simulink model "main"  (R2023b)
settings: Solver=ode113  StartTime=tstart  StopTime=tend  RelTol=relTol  AbsTol=absTol
values from neighbouring files (symbols this model uses):
  D_init = JD_init - 2451545.0    (= 1484.5)    [EulerEquations.m]    (also in main_script.m)
  DCM_initial = targetDCM([26321453.5527815,	-132781955.130633,	-57571626.5531097]', R_princ)    [EulerEquations.m]    (also in main_script.m)
  EKF_P0 = eye(7)    [main_script.m]
  EKF_x0 = [0,0,0,0,0,0,0]    [main_script.m]
  inertia_p = [85.075, 0, 0; 0, 85.075, 0; 0, 0, 120.2515]    [omega_dot.m]
  omega_init = [0; 0; 0.01]    [EulerEquations.m]    (also in main_script.m = [0; 0; 0.0])
  state_ECI_init = [R_PQW_IJK*state_PQW_init(1:3)';R_PQW_IJK*state_PQW_init(4:6)']    [OrbitPropagation.m]
  theta = UT1_to_theta(UT1)    [EulerEquations.m]    (also in UT1_to_theta.m = rotz(-GMST*180/pi); main_script.m)
  tstart = 0    [EulerEquations.m]    (also in main_script.m)
  UT1 = [1,25,2004,00]    [EulerEquations.m]    (also in main_script.m)
undefined symbols (not defined in the file or in its folder): a_sun, e_sun, i_sun, M0_sun, n_sun, Om_sun, om_sun, R_princ
libraries: dspmathops x2, aerolibatmos2 x1, simulink x1, matrix_library x1
(part 1 of 2)
settings Model: Creator=Anna  LastModifiedBy=Anna

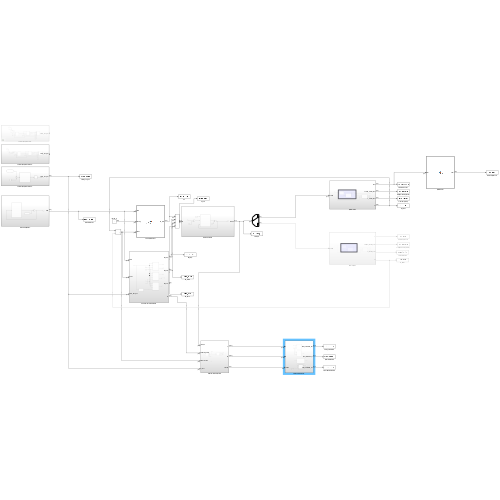
[thumbnail: Simulink's stored preview of the top-level diagram]
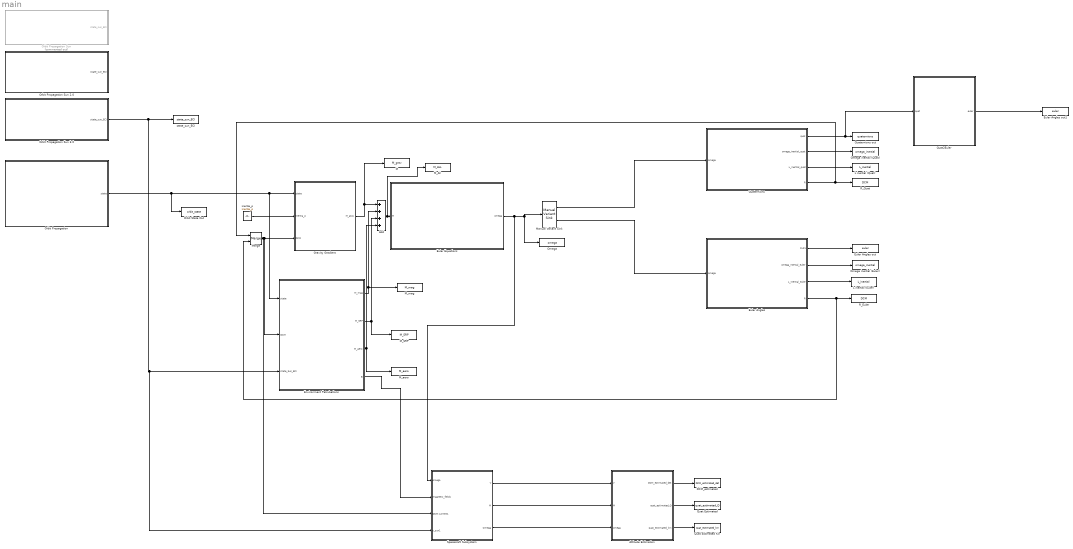
== system main ==
  Add : Sum  Inputs=++++
  Attitude Estimation : Subsystem
  DCM_estimated : ToWorkspace  VariableName=DCM_estimated_det  SaveFormat=Timeseries  SampleTime=-1
      settings: Save2DSignal=2-D array (concatenate along first dimension)
  Environment Petrubations : Subsystem
  Euler Angles : Subsystem
  Euler Angles out : ToWorkspace  VariableName=euler  SaveFormat=Timeseries  SampleTime=-1
  Euler Angles out1 : ToWorkspace  VariableName=euler  SaveFormat=Timeseries  SampleTime=-1
  Euler Equations : Subsystem
  Gravity Gradient : MATLAB Function  TreatAsAtomicUnit=on
  L inertial (Euler) : ToWorkspace  VariableName=L_inertial  SaveFormat=Timeseries  SampleTime=-1
  L inertial (Quat) : ToWorkspace  VariableName=L_inertial  SaveFormat=Timeseries  SampleTime=-1
  M : ToWorkspace  VariableName=M_grav  SaveFormat=Timeseries  SampleTime=-1
      settings: Save2DSignal=2-D array (concatenate along first dimension)
  M_All : ToWorkspace  VariableName=M_ALL  SaveFormat=Timeseries  SampleTime=-1
      settings: Save2DSignal=2-D array (concatenate along first dimension)
  M_SRP : ToWorkspace  VariableName=M_SRP  SaveFormat=Timeseries  SampleTime=-1
      settings: Save2DSignal=2-D array (concatenate along first dimension)
  M_aero : ToWorkspace  VariableName=M_aero  SaveFormat=Timeseries  SampleTime=-1
      settings: Save2DSignal=2-D array (concatenate along first dimension)
  M_mag : ToWorkspace  VariableName=M_mag  SaveFormat=Timeseries  SampleTime=-1
      settings: Save2DSignal=2-D array (concatenate along first dimension)
  Manual Variant Sink : simulink/Signal Routing/Manual Variant Sink  NumChoices=2  LabelModeActiveChoice=V_1
  Merge : Merge
  Omega : ToWorkspace  VariableName=omega  SaveFormat=Timeseries  SampleTime=-1
      settings: Save2DSignal=2-D array (concatenate along first dimension)
  Omega inertial (Euler) : ToWorkspace  VariableName=omega_inertial  SaveFormat=Timeseries  SampleTime=-1
  Omega inertial (Quat) : ToWorkspace  VariableName=omega_inertial  SaveFormat=Timeseries  SampleTime=-1
  Orbit Propagation : Subsystem
  Orbit Propagation Sun : Subsystem  Commented=on
  Orbit Propagation Sun 2.0 : Subsystem
  Orbit Propagation Sun 3.0 : Subsystem
  Orbit State Out : ToWorkspace  VariableName=orbit_state  SaveFormat=Timeseries  SampleTime=-1
  Quat Estimated : ToWorkspace  VariableName=quat_estimated_Q  SaveFormat=Timeseries  SampleTime=-1
  Quat Estimated Kin : ToWorkspace  VariableName=quat_estimated_kin  SaveFormat=Timeseries  SampleTime=-1
  Quat2Euler : MATLAB Function  TreatAsAtomicUnit=on
  Quaternions : Subsystem
  Quaternions out : ToWorkspace  VariableName=quaternions  SaveFormat=Timeseries  SampleTime=-1
  R_Euler : ToWorkspace  VariableName=DCM  SaveFormat=Timeseries  SampleTime=-1
  R_Quat : ToWorkspace  VariableName=DCM  SaveFormat=Timeseries  SampleTime=-1
  Spacecraft Subsystem : Subsystem
  inertia_p : Constant  Value=inertia_p
  state_sun_ECI : ToWorkspace  VariableName=state_sun_ECI  SaveFormat=Timeseries  SampleTime=-1
  wires:
  Quaternions/1(quat) -> Quat2Euler/1(quat), Quaternions out/1
  Quaternions/2(omega_inertial_quat) -> Omega inertial (Quat)/1
  Quaternions/3(L_inertial_quat) -> L inertial (Quat)/1
  Quaternions/4(R) -> Merge/1, R_Quat/1
  Euler Angles/1(Out1) -> Euler Angles out/1
  Euler Angles/2(omega_inertial_euler) -> Omega inertial (Euler)/1
  Euler Angles/3(L_inertial_euler) -> L inertial (Euler)/1
  Euler Angles/4(R) -> Merge/2, R_Euler/1
  Manual Variant Sink/2 -> Euler Angles/1(omega)
  Euler Equations/1(omega) -> Spacecraft Subsystem/1(omega), Manual Variant Sink/1, Omega/1
  Manual Variant Sink/1 -> Quaternions/1(omega)
  Gravity Gradient/1(M_grav) -> Add/1, M/1
  inertia_p/1 -> Gravity Gradient/2(inertia_p)
  Orbit Propagation/1(state) -> Orbit State Out/1, Gravity Gradient/1(state), Environment Petrubations/1(state)
  Quat2Euler/1(euler) -> Euler Angles out1/1
  Merge/1 -> Spacecraft Subsystem/3(DCM current1), Gravity Gradient/3(DCM), Environment Petrubations/2(DCM)
  Add/1 -> M_All/1, Euler Equations/1(M)
  Environment Petrubations/1(M_mag) -> M_mag/1, Add/2
  Environment Petrubations/2(M_SRP) -> M_SRP/1, Add/3
  Environment Petrubations/3(M_aero) -> M_aero/1, Add/4
  Orbit Propagation Sun 3.0/1(state_sun_ECI) -> state_sun_ECI/1, Environment Petrubations/3(state_Sun_ECI), Spacecraft Subsystem/4(r_sun1)
  Spacecraft Subsystem/1(V) -> Attitude Estimation/1(V)
  Spacecraft Subsystem/2(M) -> Attitude Estimation/2(M)
  Environment Petrubations/4(B) -> Spacecraft Subsystem/2(magnetic_field1)
  Attitude Estimation/1(DCM_estimated_det) -> DCM_estimated/1
  Attitude Estimation/2(quat_estimated_Q) -> Quat Estimated/1
  Attitude Estimation/3(quat_estimated_kin) -> Quat Estimated Kin/1
  Spacecraft Subsystem/3(Omega) -> Attitude Estimation/3(omega)

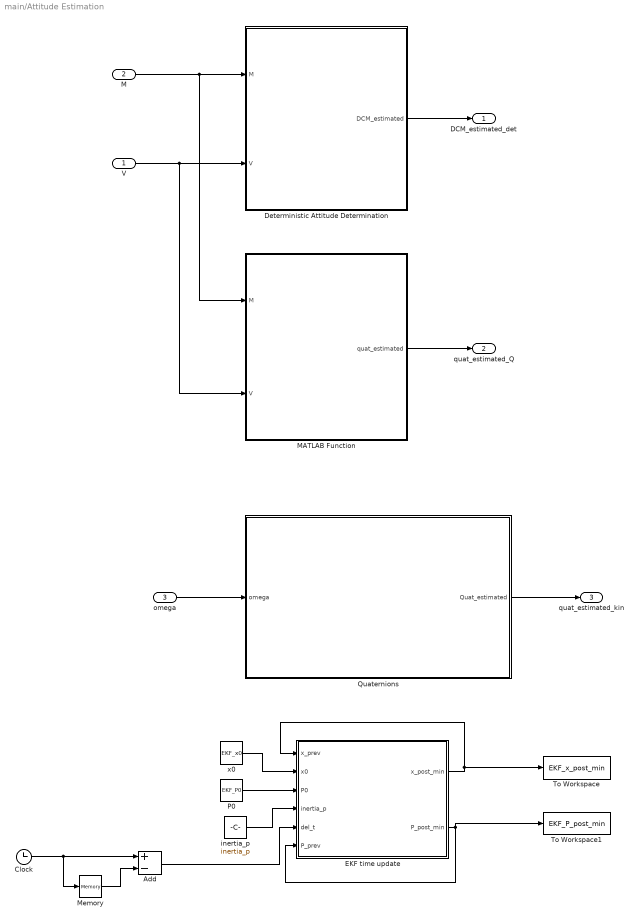
== system main/Attitude Estimation ==
  V : Inport
  M : Inport  Port=2
  omega : Inport  Port=3
  Add : Sum  Inputs=+-
  Clock : Clock
  Deterministic Attitude Determination : MATLAB Function  TreatAsAtomicUnit=on
  EKF time update : MATLAB Function  TreatAsAtomicUnit=on
  MATLAB Function : MATLAB Function  TreatAsAtomicUnit=on
  Memory : Memory
  P0 : Constant  Value=EKF_P0
  Quaternions : Subsystem
  To Workspace : ToWorkspace  VariableName=EKF_x_post_min  SaveFormat=Timeseries  SampleTime=-1
  To Workspace1 : ToWorkspace  VariableName=EKF_P_post_min  SaveFormat=Timeseries  SampleTime=-1
  inertia_p : Constant  Value=inertia_p
  x0 : Constant  Value=EKF_x0
  DCM_estimated_det : Outport
  quat_estimated_Q : Outport  Port=2
  quat_estimated_kin : Outport  Port=3
  wires:
  Deterministic Attitude Determination/1(DCM_estimated) -> DCM_estimated_det/1
  MATLAB Function/1(quat_estimated) -> quat_estimated_Q/1
  M/1 -> MATLAB Function/1(M), Deterministic Attitude Determination/1(M)
  Quaternions/1(Quat_estimated) -> quat_estimated_kin/1
  V/1 -> MATLAB Function/2(V), Deterministic Attitude Determination/2(V)
  omega/1 -> Quaternions/1(omega)
  EKF time update/1(x_post_min) -> To Workspace/1, EKF time update/1(x_prev)
  EKF time update/2(P_post_min) -> To Workspace1/1, EKF time update/6(P_prev)
  x0/1 -> EKF time update/2(x0)
  P0/1 -> EKF time update/3(P0)
  inertia_p/1 -> EKF time update/4(inertia_p)
  Add/1 -> EKF time update/5(del_t)
  Memory/1 -> Add/2
  Clock/1 -> Memory/1, Add/1

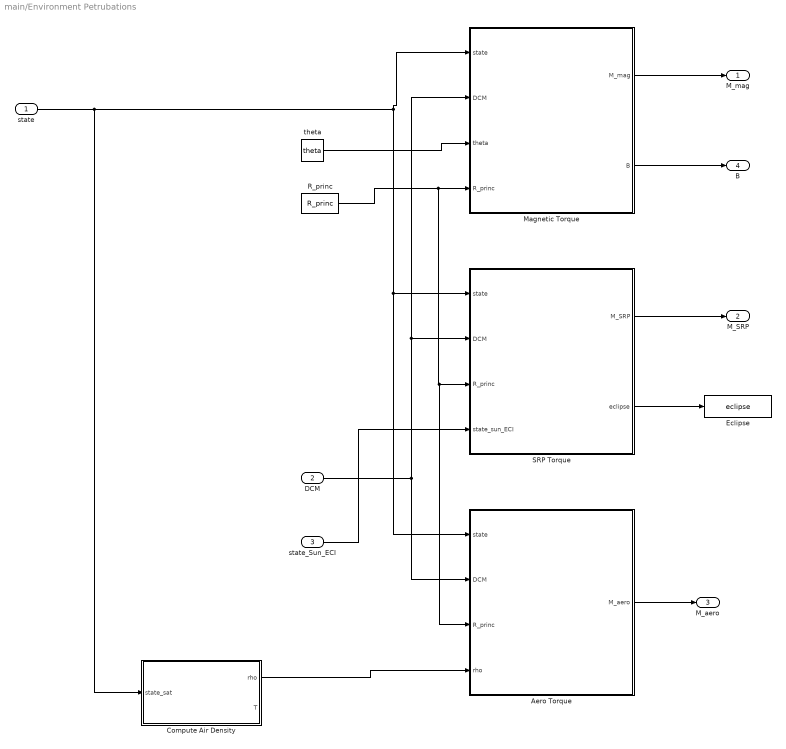
== system main/Environment Petrubations ==
  state : Inport
  DCM : Inport  Port=2
  state_Sun_ECI : Inport  Port=3
  Aero Torque : MATLAB Function  TreatAsAtomicUnit=on
  Compute Air Density : Subsystem
  Eclipse : ToWorkspace  VariableName=eclipse  SaveFormat=Timeseries  SampleTime=-1
  Magnetic Torque : MATLAB Function  TreatAsAtomicUnit=on
  R_princ : Constant  Value=R_princ
  SRP Torque : MATLAB Function  TreatAsAtomicUnit=on
  theta : Constant  Value=theta
  M_mag : Outport
  M_SRP : Outport  Port=2
  M_aero : Outport  Port=3
  B : Outport  Port=4
  wires:
  Magnetic Torque/1(M_mag) -> M_mag/1
  SRP Torque/1(M_SRP) -> M_SRP/1
  state/1 -> Compute Air Density/1(state_sat), Magnetic Torque/1(state), Aero Torque/1(state), SRP Torque/1(state)
  DCM/1 -> Aero Torque/2(DCM), Magnetic Torque/2(DCM), SRP Torque/2(DCM)
  theta/1 -> Magnetic Torque/3(theta)
  R_princ/1 -> Aero Torque/3(R_princ), SRP Torque/3(R_princ), Magnetic Torque/4(R_princ)
  state_Sun_ECI/1 -> SRP Torque/4(state_sun_ECI)
  Aero Torque/1(M_aero) -> M_aero/1
  Compute Air Density/1(rho) -> Aero Torque/4(rho)
  SRP Torque/2(eclipse) -> Eclipse/1
  Magnetic Torque/2(B) -> B/1

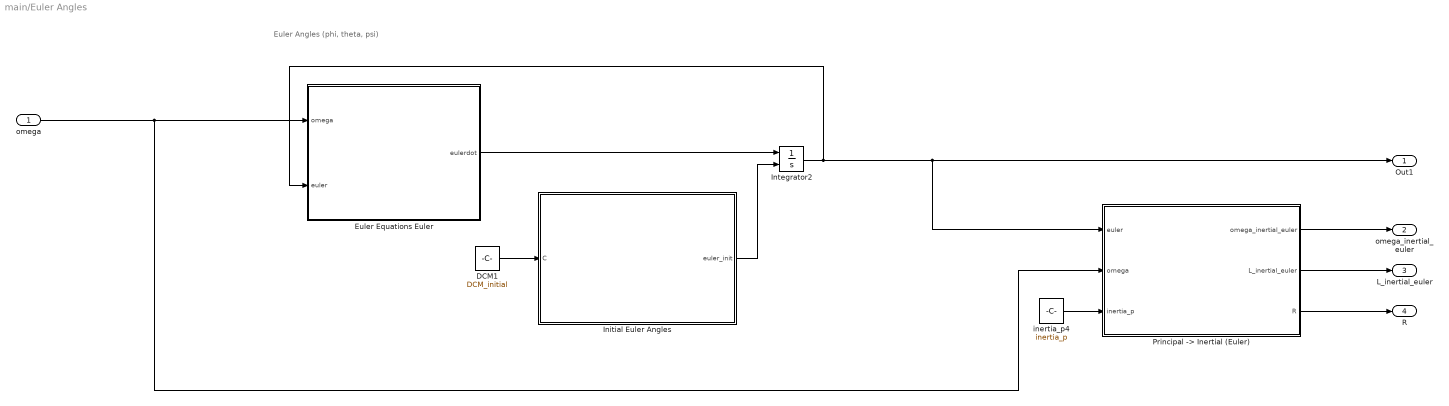
== system main/Euler Angles ==
  note: Euler Angles (phi, theta, psi)
  omega : Inport
  DCM1 : Constant  Value=DCM_initial
  Euler Equations Euler : MATLAB Function  TreatAsAtomicUnit=on
  Initial Euler Angles : MATLAB Function  TreatAsAtomicUnit=on
  Integrator2 : Integrator  InitialConditionSource=external  AbsoluteTolerance=absTol
  "Principal -> Inertial (Euler)" : MATLAB Function  TreatAsAtomicUnit=on
  inertia_p4 : Constant  Value=inertia_p
  Out1 : Outport
  omega_inertial_euler : Outport  Port=2
  L_inertial_euler : Outport  Port=3
  R : Outport  Port=4
  wires:
  "Principal -> Inertial (Euler)"/2(L_inertial_euler) -> L_inertial_euler/1
  Initial Euler Angles/1(euler_init) -> Integrator2/2
  "Principal -> Inertial (Euler)"/1(omega_inertial_euler) -> omega_inertial_euler/1
  "Principal -> Inertial (Euler)"/3(R) -> R/1
  Integrator2/1 -> Out1/1, "Principal -> Inertial (Euler)"/1(euler), Euler Equations Euler/2(euler)
  Euler Equations Euler/1(eulerdot) -> Integrator2/1
  omega/1 -> "Principal -> Inertial (Euler)"/2(omega), Euler Equations Euler/1(omega)
  inertia_p4/1 -> "Principal -> Inertial (Euler)"/3(inertia_p)
  DCM1/1 -> Initial Euler Angles/1(C)

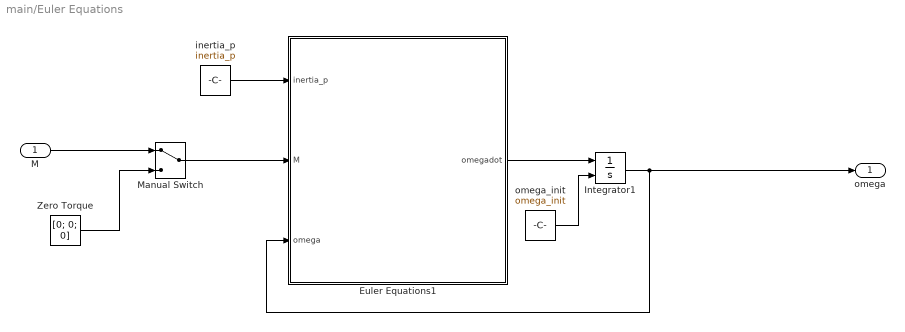
== system main/Euler Equations ==
  M : Inport
  Euler Equations1 : MATLAB Function  TreatAsAtomicUnit=on
  Integrator1 : Integrator  InitialConditionSource=external  AbsoluteTolerance=absTol
  Manual Switch : ManualSwitch
  Zero Torque : Constant  Value=[0; 0; 0]
  inertia_p : Constant  Value=inertia_p
  omega_init : Constant  Value=omega_init
  omega : Outport
  wires:
  inertia_p/1 -> Euler Equations1/1(inertia_p)
  Euler Equations1/1(omegadot) -> Integrator1/1
  Integrator1/1 -> omega/1, Euler Equations1/3(omega)
  omega_init/1 -> Integrator1/2
  Manual Switch/1 -> Euler Equations1/2(M)
  M/1 -> Manual Switch/1
  Zero Torque/1 -> Manual Switch/2

== system main/Orbit Propagation ==
  Integrator3 : Integrator  InitialConditionSource=external  AbsoluteTolerance=absTol
  Orbit Propagation1 : MATLAB Function  TreatAsAtomicUnit=on
  initial state ECI : Constant  Value=state_ECI_init
  state : Outport
  wires:
  initial state ECI/1 -> Integrator3/2
  Orbit Propagation1/1(statedot) -> Integrator3/1
  Integrator3/1 -> state/1, Orbit Propagation1/1(state)

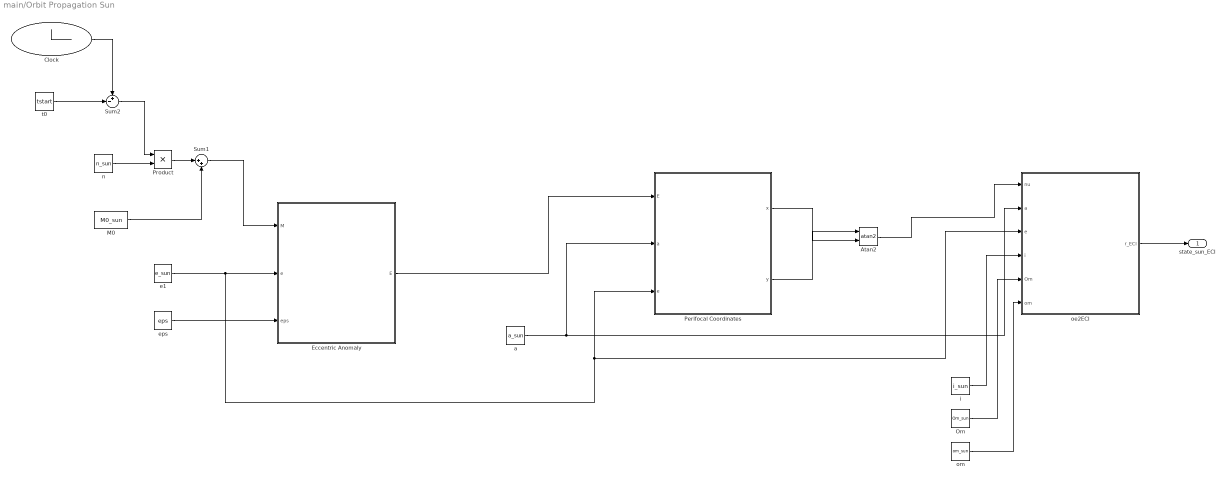
== system main/Orbit Propagation Sun ==
  Atan2 : Trigonometry  Operator=atan2
  Clock : Clock
  Eccentric Anomaly : MATLAB Function  TreatAsAtomicUnit=on
  M0 : Constant  Value=M0_sun
  Om : Constant  Value=Om_sun
  Perifocal Coordinates : MATLAB Function  TreatAsAtomicUnit=on
  Product : Product
  Sum1 : Sum  Inputs=|++
  Sum2 : Sum  Inputs=+-|
  a : Constant  Value=a_sun
  e1 : Constant  Value=e_sun
  eps : Constant  Value=eps
  i : Constant  Value=i_sun
  n : Constant  Value=n_sun
  oe2ECI : MATLAB Function  TreatAsAtomicUnit=on
  om : Constant  Value=om_sun
  t0 : Constant  Value=tstart
  state_sun_ECI : Outport
  wires:
  oe2ECI/1(r_ECI) -> state_sun_ECI/1
  Om/1 -> oe2ECI/5(Om)
  Perifocal Coordinates/2(y) -> Atan2/1
  Perifocal Coordinates/1(x) -> Atan2/2
  i/1 -> oe2ECI/4(i)
  Atan2/1 -> oe2ECI/1(nu)
  e1/1 -> oe2ECI/3(e), Perifocal Coordinates/3(e), Eccentric Anomaly/2(e)
  a/1 -> Perifocal Coordinates/2(a), oe2ECI/2(a)
  om/1 -> oe2ECI/6(om)
  eps/1 -> Eccentric Anomaly/3(eps)
  Eccentric Anomaly/1(E) -> Perifocal Coordinates/1(E)
  Sum1/1 -> Eccentric Anomaly/1(M)
  M0/1 -> Sum1/2
  Sum2/1 -> Product/1
  Clock/1 -> Sum2/1
  n/1 -> Product/2
  Product/1 -> Sum1/1
  t0/1 -> Sum2/2

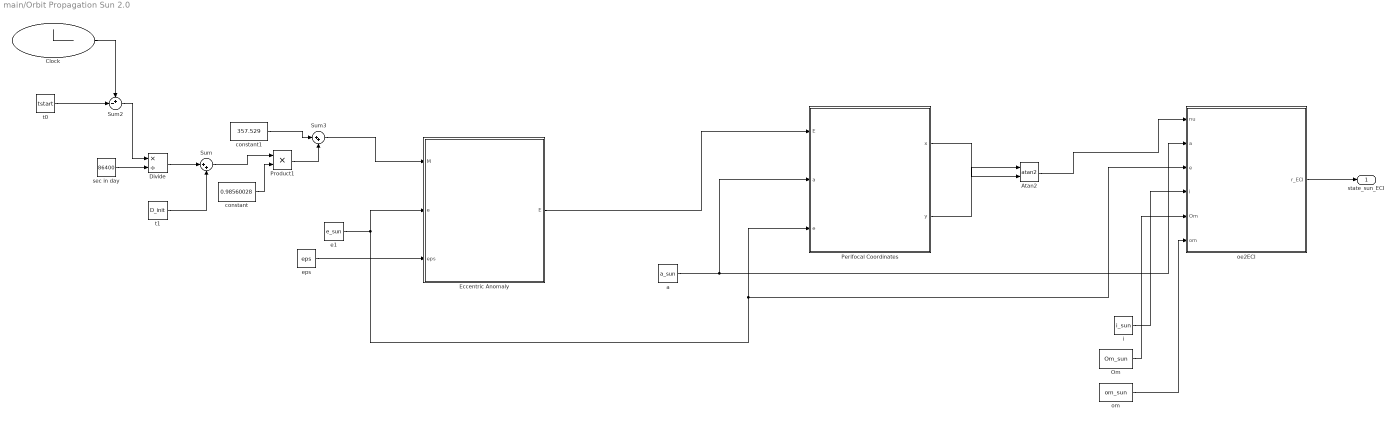
== system main/Orbit Propagation Sun 2.0 ==
  Atan2 : Trigonometry  Operator=atan2
  Clock : Clock
  Divide : Product  Inputs=*/
  Eccentric Anomaly : MATLAB Function  TreatAsAtomicUnit=on
  Om : Constant  Value=Om_sun
  Perifocal Coordinates : MATLAB Function  TreatAsAtomicUnit=on
  Product1 : Product
  Sum : Sum  Inputs=|++
  Sum2 : Sum  Inputs=+-|
  Sum3 : Sum  Inputs=|++
  a : Constant  Value=a_sun
  constant : Constant  Value=0.98560028
  constant1 : Constant  Value=357.529
  e1 : Constant  Value=e_sun
  eps : Constant  Value=eps
  i : Constant  Value=i_sun
  oe2ECI : MATLAB Function  TreatAsAtomicUnit=on
  om : Constant  Value=om_sun
  sec in day : Constant  Value=86400
  t0 : Constant  Value=tstart
  t1 : Constant  Value=D_init
  state_sun_ECI : Outport
  wires:
  oe2ECI/1(r_ECI) -> state_sun_ECI/1
  Om/1 -> oe2ECI/5(Om)
  Perifocal Coordinates/2(y) -> Atan2/1
  Perifocal Coordinates/1(x) -> Atan2/2
  i/1 -> oe2ECI/4(i)
  Atan2/1 -> oe2ECI/1(nu)
  e1/1 -> Eccentric Anomaly/2(e), oe2ECI/3(e), Perifocal Coordinates/3(e)
  a/1 -> Perifocal Coordinates/2(a), oe2ECI/2(a)
  om/1 -> oe2ECI/6(om)
  eps/1 -> Eccentric Anomaly/3(eps)
  Eccentric Anomaly/1(E) -> Perifocal Coordinates/1(E)
  Clock/1 -> Sum2/1
  t0/1 -> Sum2/2
  Sum2/1 -> Divide/1
  sec in day/1 -> Divide/2
  Divide/1 -> Sum/1
  t1/1 -> Sum/2
  Sum/1 -> Product1/1
  constant/1 -> Product1/2
  Product1/1 -> Sum3/2
  constant1/1 -> Sum3/1
  Sum3/1 -> Eccentric Anomaly/1(M)

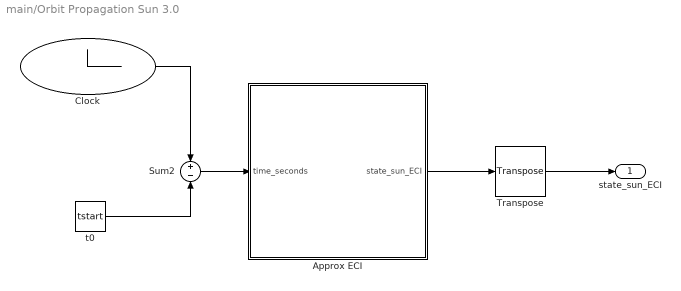
== system main/Orbit Propagation Sun 3.0 ==
  Approx ECI : MATLAB Function  TreatAsAtomicUnit=on
  Clock : Clock
  Sum2 : Sum  Inputs=+-
  Transpose : matrix_library/Transpose
  t0 : Constant  Value=tstart
  state_sun_ECI : Outport
  wires:
  Clock/1 -> Sum2/1
  t0/1 -> Sum2/2
  Sum2/1 -> Approx ECI/1(time_seconds)
  Transpose/1 -> state_sun_ECI/1
  Approx ECI/1(state_sun_ECI) -> Transpose/1

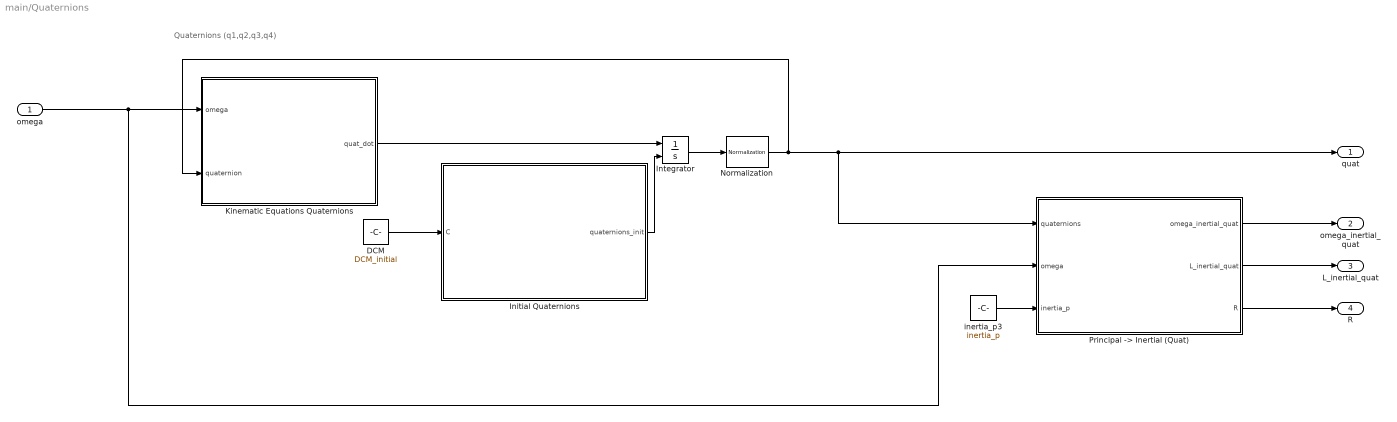
== system main/Quaternions ==
  note: Quaternions (q1,q2,q3,q4)
  omega : Inport
  DCM : Constant  Value=DCM_initial
  Initial Quaternions : MATLAB Function  TreatAsAtomicUnit=on
  Integrator : Integrator  InitialConditionSource=external  AbsoluteTolerance=absTol
  "Kinematic Equations Quaternions " : MATLAB Function  TreatAsAtomicUnit=on
  Normalization : dspmathops/Normalization  NormType=Squared 2-norm  Bias=1e-10  NormOver=Each column  Dimension=1  roundingMode=Floor  overflowMode=off  accumDataTypeStr=Inherit: Same as product output  accumLastDataTypeStr=Inherit: Same as product output  outputDataTypeStr=Inherit: Same as product output  outputMin=[]  outputMax=[]  outputLastDataTypeStr=Inherit: Same as product output
  "Principal -> Inertial (Quat)" : MATLAB Function  TreatAsAtomicUnit=on
  inertia_p3 : Constant  Value=inertia_p
  quat : Outport
  omega_inertial_quat : Outport  Port=2
  L_inertial_quat : Outport  Port=3
  R : Outport  Port=4
  wires:
  omega/1 -> "Kinematic Equations Quaternions "/1(omega), "Principal -> Inertial (Quat)"/2(omega)
  DCM/1 -> Initial Quaternions/1(C)
  "Principal -> Inertial (Quat)"/2(L_inertial_quat) -> L_inertial_quat/1
  "Kinematic Equations Quaternions "/1(quat_dot) -> Integrator/1
  "Principal -> Inertial (Quat)"/3(R) -> R/1
  Initial Quaternions/1(quaternions_init) -> Integrator/2
  Integrator/1 -> Normalization/1
  inertia_p3/1 -> "Principal -> Inertial (Quat)"/3(inertia_p)
  "Principal -> Inertial (Quat)"/1(omega_inertial_quat) -> omega_inertial_quat/1
  Normalization/1 -> quat/1, "Principal -> Inertial (Quat)"/1(quaternions), "Kinematic Equations Quaternions "/2(quaternion)

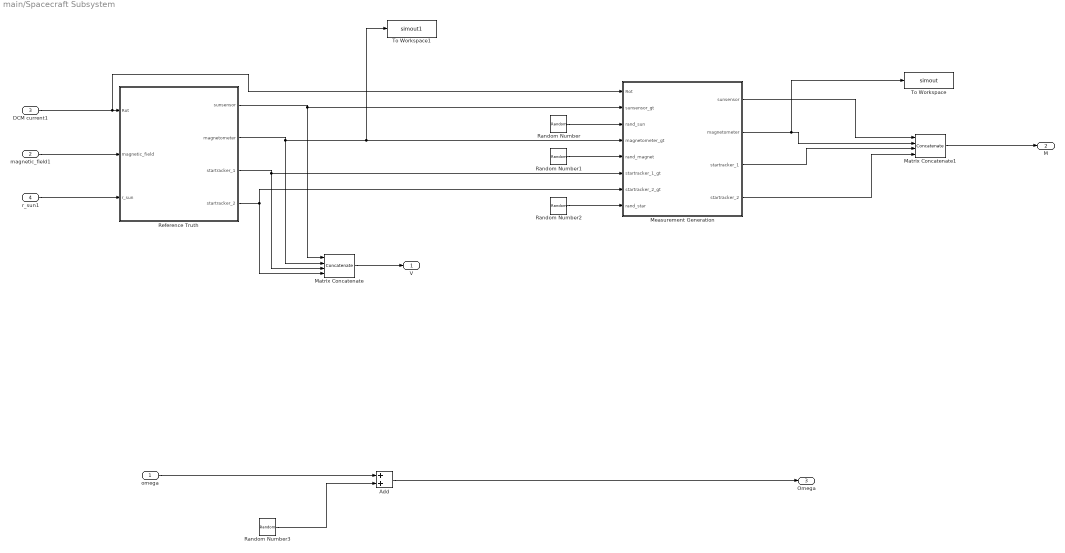
== system main/Spacecraft Subsystem ==
  omega : Inport
  magnetic_field1 : Inport  Port=2
  DCM current1 : Inport  Port=3
  r_sun1 : Inport  Port=4
  Add : Sum
  Matrix Concatenate : Concatenate  NumInputs=4  Mode=Multidimensional array  ConcatenateDimension=2
  Matrix Concatenate1 : Concatenate  NumInputs=4  Mode=Multidimensional array  ConcatenateDimension=2
  Measurement Generation : MATLAB Function  TreatAsAtomicUnit=on
  Random Number : RandomNumber  Variance=0.01  Seed=[80, 81]  SampleTime=0.1
  Random Number1 : RandomNumber  Variance=0.0075*0.000065  Seed=[70, 71, 72]  SampleTime=0.1
  Random Number2 : RandomNumber  Variance=(5/3600)  Seed=[0, 1,2,3,4,5,6,7,8,9,10,11,12,13,14; 15,16,17,18,19,20,21,22,23,24,25,26,27,28,29; 30, 31, 32,33,34,35,36,37,38,39,40,41,42,43,44;45,46,47,48,49,50,51,52,53,54,55,56,57,58,59]  SampleTime=0.1
  Random Number3 : RandomNumber  Variance=0.005  Seed=[101, 102, 103]  SampleTime=0.1
  Reference Truth : MATLAB Function  TreatAsAtomicUnit=on
  To Workspace : ToWorkspace  VariableName=simout  SaveFormat=Timeseries  SampleTime=-1
  To Workspace1 : ToWorkspace  VariableName=simout1  SaveFormat=Timeseries  SampleTime=-1
  V : Outport
  M : Outport  Port=2
  Omega : Outport  Port=3
  wires:
  r_sun1/1 -> Reference Truth/3(r_sun)
  magnetic_field1/1 -> Reference Truth/2(magnetic_field)
  DCM current1/1 -> Measurement Generation/1(Rot), Reference Truth/1(Rot)
  Matrix Concatenate1/1 -> M/1
  Matrix Concatenate/1 -> V/1
  Reference Truth/1(sunsensor) -> Matrix Concatenate/1, Measurement Generation/2(sunsensor_gt)
  Reference Truth/3(startracker_1) -> Measurement Generation/6(startracker_1_gt), Matrix Concatenate/3
  Reference Truth/4(startracker_2) -> Measurement Generation/7(startracker_2_gt), Matrix Concatenate/4
  Measurement Generation/1(sunsensor) -> Matrix Concatenate1/1
  Random Number/1 -> Measurement Generation/3(rand_sun)
  Random Number1/1 -> Measurement Generation/5(rand_magnet)
  Random Number2/1 -> Measurement Generation/8(rand_star)
  Measurement Generation/2(magnetometer) -> To Workspace/1, Matrix Concatenate1/2
  Measurement Generation/4(startracker_2) -> Matrix Concatenate1/4
  Reference Truth/2(magnetometer) -> To Workspace1/1, Measurement Generation/4(magnetometer_gt), Matrix Concatenate/2
  Measurement Generation/3(startracker_1) -> Matrix Concatenate1/3
  omega/1 -> Add/1
  Random Number3/1 -> Add/2
  Add/1 -> Omega/1

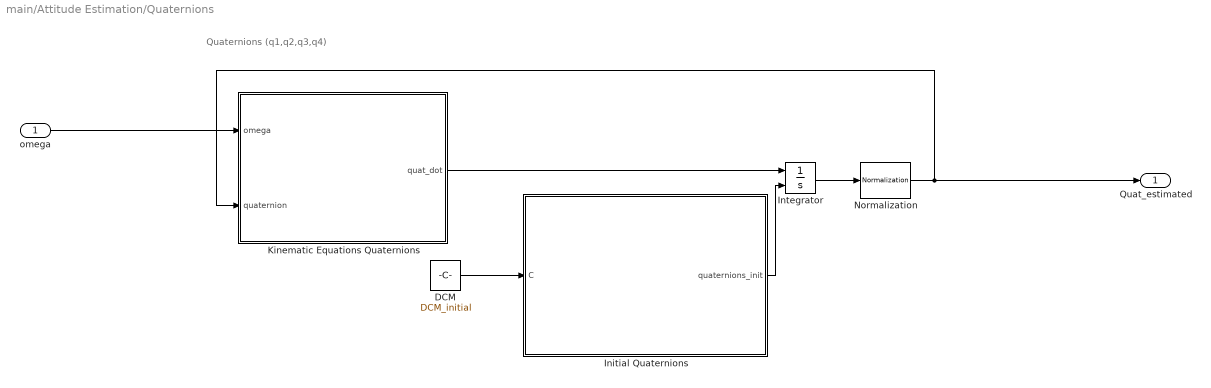
== system main/Attitude Estimation/Quaternions ==
  note: Quaternions (q1,q2,q3,q4)
  omega : Inport
  DCM : Constant  Value=DCM_initial
  Initial Quaternions : MATLAB Function  TreatAsAtomicUnit=on
  Integrator : Integrator  InitialConditionSource=external  AbsoluteTolerance=absTol
  "Kinematic Equations Quaternions " : MATLAB Function  TreatAsAtomicUnit=on
  Normalization : dspmathops/Normalization  NormType=Squared 2-norm  Bias=1e-10  NormOver=Each column  Dimension=1  roundingMode=Floor  overflowMode=off  accumDataTypeStr=Inherit: Same as product output  accumLastDataTypeStr=Inherit: Same as product output  outputDataTypeStr=Inherit: Same as product output  outputMin=[]  outputMax=[]  outputLastDataTypeStr=Inherit: Same as product output
  Quat_estimated : Outport
  wires:
  omega/1 -> "Kinematic Equations Quaternions "/1(omega)
  DCM/1 -> Initial Quaternions/1(C)
  "Kinematic Equations Quaternions "/1(quat_dot) -> Integrator/1
  Initial Quaternions/1(quaternions_init) -> Integrator/2
  Integrator/1 -> Normalization/1
  Normalization/1 -> Quat_estimated/1, "Kinematic Equations Quaternions "/2(quaternion)

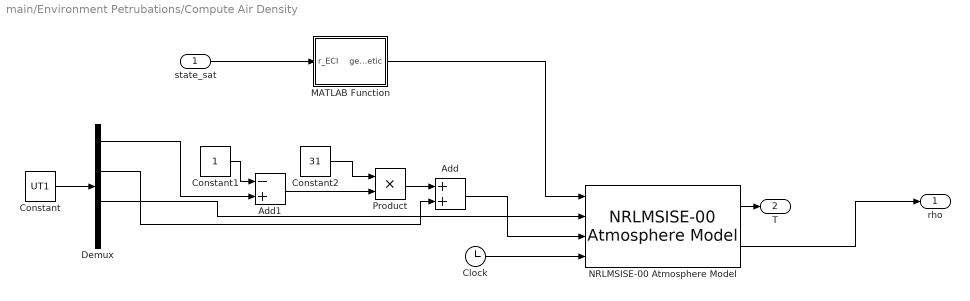
== system main/Environment Petrubations/Compute Air Density ==
  state_sat : Inport
  Add : Sum
  Add1 : Sum  Inputs=-+
  Clock : Clock
  Constant : Constant  Value=UT1
  Constant1 : Constant
  Constant2 : Constant  Value=31
  Demux : Demux
  MATLAB Function : MATLAB Function  TreatAsAtomicUnit=on
  NRLMSISE-00 Atmosphere Model : aerolibatmos2/NRLMSISE-00 Atmosphere Model  units=Metric (MKS)  lst_input=off  flux_ap_input=off  flags_input=Internal  flags=ones(1,23)  oxygen_in=off  action=Warning
  Product : Product
  rho : Outport
  T : Outport  Port=2
  wires:
  NRLMSISE-00 Atmosphere Model/1 -> T/1
  Demux/2 -> Add/2
  NRLMSISE-00 Atmosphere Model/2 -> rho/1
  Product/1 -> Add/1
  Add/1 -> NRLMSISE-00 Atmosphere Model/3
  MATLAB Function/1(geodetic) -> NRLMSISE-00 Atmosphere Model/1
  Demux/1 -> Add1/2
  Demux/3 -> NRLMSISE-00 Atmosphere Model/2
  Clock/1 -> NRLMSISE-00 Atmosphere Model/4
  Add1/1 -> Product/2
  Constant/1 -> Demux/1
  Constant2/1 -> Product/1
  state_sat/1 -> MATLAB Function/1(r_ECI)
  Constant1/1 -> Add1/1

== matlab function main/Gravity Gradient ==
  data: state input; inertia_p input; DCM input; M_grav output
%% return omega_dot (zero torque)
function M_grav  = gravity_gradient(state, inertia_p, DCM)
    mu = 398600.435436; %Earth centered orbit

    R_p = DCM * state(1:3);
    cx = R_p(1)/norm(R_p);
    cy = R_p(2)/norm(R_p);
    cz = R_p(3)/norm(R_p);

    M_grav = 3*mu/(norm(R_p)^3) *[(inertia_p(3,3) - inertia_p(2,2)) * cy * cz;
                    (inertia_p(1,1) - inertia_p(3,3)) * cz * cx;
                    (inertia_p(2,2) - inertia_p(1,1)) * cx * cy];
 
 
    %disp(norm(M))
end

== matlab function main/Quat2Euler ==
  data: quat input; euler output

%% return euler angles from quaternions
function euler= quat2eul(quat)
    q0 = quat(4);
    q1 = quat(1);
    q2 = quat(2);
    q3 = quat(3);

    %123 singular for theta = 90 deg
    %phi = atan2(2*q2*q3 + 2*q0*q1, q3^2 - q2^2 - q1^2 + q0^2);
    %theta = -asin(2*q1*q3 - 2*q0*q2);
    %psi = atan2(2*q1*q2 + 2*q0*q3, q1^2 + q0^2 - q3^2 - q2^2);

    % %213 use when you rotate around y, singular for theta = 90
    phi = atan2(-2*q1*q3 + 2*q0*q2, q3^2 - q2^2 - q1^2 + q0^2);
    theta = asin(2*q2*q3 + 2*q0*q1);
    psi = atan2(-2*q1*q2 + 2*q0*q3, q2^2 - q3^2 + q0^2 - q1^2);

    %313 singular for theta = 0
    %phi = atan2(2*q1*q3 - 2*q0*q2, 2*q2*q3 + 2*q0*q1);
    %theta = acos(q3^2 - q2^2 - q1^2 + q0^2);
    %psi =atan2(2*q1*q3 + 2*q0*q2, -2*q2*q3 + 2*q0*q1);
    
    euler = [phi; theta; psi];

end

== matlab function main/Orbit Propagation Sun/Eccentric Anomaly ==
  data: M input; E output; e input; eps input
function E = eccentric_anomaly(M, e, eps)
    delta = 2*eps;
    E_i = M;
    E = 2*M;
    while delta > eps
        E = E_i - (E_i - e * sin(E_i) - M)/(1 - e*cos(E_i));
        delta = abs(E - E_i);
        E_i = E;
    end
end

== matlab function main/Orbit Propagation Sun/Perifocal Coordinates ==
  data: E input; x output; y output; a input; e input
function [x,y] = perifocal_coords(E, a, e)
    x = a*(cos(E) - e);
    y = a * sqrt(1 - e^2) * sin(E);
end

== matlab function main/Orbit Propagation Sun/oe2ECI ==
  data: nu input; a input; e input; i input; r_ECI output; Om input; om input
function r_ECI =   OE2ECI(nu, a, e, i, Om, om)
    %mu = 398600.435507;

    Rot_Om = [cosd(-Om) sind(-Om) 0;
              -sind(-Om) cosd(-Om) 0
              0 0 1];
    Rot_i = [1 0 0;
            0 cosd(-i) sind(-i);
            0 -sind(-i) cosd(-i)];
    Rot_om = [cosd(-om) sind(-om) 0;
              -sind(-om) cosd(-om) 0
              0 0 1];
    R = Rot_Om * Rot_i * Rot_om;

    
    % Position    
    p = a*(1-e^2);
    r = p/(1+e*cos(nu));
    r_ECI = R * [r*cos(nu); r*sin(nu); 0]; %position vector

end

== matlab function main/Environment Petrubations/SRP Torque ==
  data: state input; DCM input; R_princ input; M_SRP output; state_sun_ECI input; eclipse output
function [M_SRP, eclipse] = SRP_torque(state, DCM, R_princ, state_sun_ECI)
    P = 1358/(3e8); % Solar Constant

    R = state(1:3)*1000; % State ECI
    R_unit = R./norm(R); % Unit State ECI
    R_E = 6378*1000; % Earth Radius

    R_Sun = state_sun_ECI; % Sun State ECI 
    R_Sun_unit = R_Sun./norm(R_Sun); % Unit Sun State ECI
    R_p_Sun = DCM * R_Sun; % Sun State Princ
    R_p_Sun_unit = R_p_Sun./norm(R_p_Sun); % Unit Sun State Princ

    M_SRP = [0;0;0];

    surface = struct('bary',[0,0,0],'size',0,'unit',[0,0,0]);

    % Eclipses
    psi = acos(dot(R_unit, R_Sun_unit));
    a_check = norm(R)*sin(psi);

    for surfacenum = 1:20
        if surfacenum == 1
            surface.bary = [-0.0129, -0.0019, 1.0022]; % Converted from cm to m
            surface.size = 0.866025; % Converted from cm² to m²
            surface.unit = [0, 0, 1];
        end
        if surfacenum == 2
            surface.bary = [-0.0129, -0.0019, -0.6008]; % Converted from cm to m
            surface.size = 0.866025; % Converted from cm² to m²
            surface.unit = [0, 0, -1];
        end
        if surfacenum == 3
            surface.bary = [0.4871, -0.0019, 0.2007]; % Converted from cm to m
            surface.size = 0.913944; % Converted from cm² to m²
            surface.unit = [1, 0, 0];
        end
        if surfacenum == 4
            surface.bary = [1.0854, -0.0019, -0.5808]; % Converted from cm to m
            surface.size = 0.690859; % Converted from cm² to m²
            surface.unit = [0, 0, 1];
        end
        if surfacenum == 5
            surface.bary = [1.0854, -0.0019, -0.6008]; % Converted from cm to m
            surface.size = 0.690859; % Converted from cm² to m²
            surface.unit = [0, 0, -1];
        end
        if surfacenum == 6
            surface.bary = [0.2371, 0.4311, 0.2007]; % Converted from cm to m
            surface.size = 0.913944; % Converted from cm² to m²
            surface.unit = [0.5, 0.866, 0];
        end
        if surfacenum == 7
            surface.bary = [0.5362, 0.9492, -0.5808]; % Converted from cm to m
            surface.size = 0.690859; % Converted from cm² to m²
            surface.unit = [0, 0, 1];
        end
        if surfacenum == 8
            surface.bary = [0.5362, 0.9492, -0.6008]; % Converted from cm to m
            surface.size = 0.690859; % Converted from cm² to m²
            surface.unit = [0, 0, -1];
        end
        if surfacenum == 9
            surface.bary = [-0.2629, 0.4311, 0.2007]; % Converted from cm to m
            surface.size = 0.913944; % Converted from cm² to m²
            surface.unit = [-0.5, 0.866, 0];
        end
        if surfacenum == 10
            surface.bary = [-0.5620, 0.9492, -0.5808]; % Converted from cm to m
            surface.size = 0.690859; % Converted from cm² to m²
            surface.unit = [0, 0, 1];
        end
        if surfacenum == 11
            surface.bary = [-0.5620, 0.9492, -0.6008]; % Converted from cm to m
            surface.size = 0.690859; % Converted from cm² to m²
            surface.unit = [0, 0, -1];
        end
        if surfacenum == 12
            surface.bary = [-0.5129, -0.0019, 0.2007]; % Converted from cm to m
            surface.size = 0.913944; % Converted from cm² to m²
            surface.unit = [-1, 0, 0];
        end
        if surfacenum == 13
            surface.bary = [-1.1111, -0.0019, -0.5808]; % Converted from cm to m
            surface.size = 0.690859; % Converted from cm² to m²
            surface.unit = [0, 0, 1];
        end
        if surfacenum == 14
            surface.bary = [-1.1111, -0.0019, -0.6008]; % Converted from cm to m
            surface.size = 0.690859; % Converted from cm² to m²
            surface.unit = [0, 0, -1];
        end
        if surfacenum == 15
            surface.bary = [-0.2629, -0.4349, 0.2007]; % Converted from cm to m
            surface.size = 0.913944; % Converted from cm² to m²
            surface.unit = [-0.5, -0.866, 0];
        end
        if surfacenum == 16
            surface.bary = [-0.5620, -0.9530, -0.5808]; % Converted from cm to m
            surface.size = 0.690859; % Converted from cm² to m²
            surface.unit = [0, 0, 1];
        end
        if surfacenum == 17
            surface.bary = [-0.5620, -0.9530, -0.6008]; % Converted from cm to m
            surface.size = 0.690859; % Converted from cm² to m²
            surface.unit = [0, 0, -1];
        end
        if surfacenum == 18
            surface.bary = [0.2371, -0.4349, 0.2007]; % Converted from cm to m
            surface.size = 0.913944; % Converted from cm² to m²
            surface.unit = [0.5, -0.866, 0];
        end
        if surfacenum == 19
            surface.bary = [0.5362, -0.9530, -0.5808]; % Converted from cm to m
            surface.size = 0.690859; % Converted from cm² to m²
            surface.unit = [0, 0, 1];
        end
        if surfacenum == 20
            surface.bary = [0.5362, -0.9530, -0.6008]; % Converted from cm to m
            surface.size = 0.690859; % Converted from cm² to m²
            surface.unit = [0, 0, -1];
        end

        bary = R_princ*(surface.bary'); % Barycenter body to princ
        A = (surface.size); % Area in m^2
        N = R_princ*(surface.unit'); % Normal vector in princ
        
        %cos_theta_StoN = dot(N,R_p_Sun_unit); % Angle between N and S vectors
        theta_StoN = acos(dot(N, R_p_Sun_unit));
        
        C_s = 0.7; % Aluminum about 70% specular reflectance 
        C_d = 0.15; 
        % 
        % disp(theta_StoN)
        % % Check if the angle is within the range of 0 to 90 degrees
        if theta_StoN >= 0 && theta_StoN <= pi/2
            e = 1; % Surfaces can see each other
        else
            e = 0; % Surfaces are obstructed
        end
        % 
        F = -P*A*cos(theta_StoN) * ((1-C_s)*R_p_Sun_unit + 2*(C_s*cos(theta_StoN) + (1/3)*C_d)*N); % Force

        M_SRP = M_SRP + e*cross(bary,F); % Summation 
    end
    eclipse = 0;
    if a_check < R_E && psi > pi/2
        eclipse = 1;
        M_SRP = [0;0;0];
    end
end

== matlab function main/Environment Petrubations/Magnetic Torque ==
  data: state input; DCM input; theta input; M_mag output; R_princ input; B output
%% return omega_dot (zero torque)
function [M_mag, B] = mag_torque(state, DCM, theta, R_princ)
    eps = 4*pi*10^-7; % Vacuum Perm
    S = 0.866025; % Surface Area inside coils, m^2
    n = 100; % Coils
    I = 35.4/25; % Current, Power/Voltage for SIM

    R = state(1:3)*1000; % State
    R_unit = R/norm(R); % Unit State
    R_E = 6378*1000; % Earth Radius
    R_p = DCM * R; % Attitude

    % Earth Mag Dipole Point Lat Long Initial
    lambda = -115.62;
    phi = 82.752;

    m_initial = R_E*[cosd(phi)*cosd(lambda);cosd(phi)*sind(lambda);sind(phi)]; % In ECEF
    m_initial = m_initial./norm(m_initial);

    m = theta*m_initial; % ECEF to ECI
    m = DCM*m; % ECI to Current Principal
    B_0 = 3.08e-5; % Earth Dipole Strength, Teslas
    
    m_sat = R_princ*[0,0,1]'; % Body to Current Principal
    m_sat = eps*S*n*I*m_sat'; % Satellite Mag Moment
    B = -((R_E^3)*B_0/(norm(R)^3)) * (3*(dot(m,R_unit))*R_unit - m); % Earth Mag Field Inertial

    M_mag = cross(m_sat,B)'; % Mag Moment
end

== matlab function main/Environment Petrubations/Aero Torque ==
  data: state input; DCM input; R_princ input; M_aero output; rho input
function M_aero = aero_torque(state, DCM, R_princ, rho)
    V = state(4:6)*1000; % Satellite Velocity
    V_p = DCM * V; % In Principal
    V_p_unit = V_p./norm(V_p); % Velocity Norm in princ

    C_d = 1.28; % Flat Plates
    % h = norm(R) - R_E; % Satellite height in meters
    % rho = 1.454*10^(-13); %(1.45e-4) * exp(-(h - 6e2) ./ 7.1835e1)
    M_aero = [0;0;0];

    rho = rho(6);

    surface = struct('bary',[0,0,0],'size',0,'unit',[0,0,0]);

    for surfacenum = 1:20
        if surfacenum == 1
            surface.bary = [-0.0129, -0.0019, 1.0022]; % Converted from cm to m
            surface.size = 0.866025; % Converted from cm² to m²
            surface.unit = [0, 0, 1];
        end
        if surfacenum == 2
            surface.bary = [-0.0129, -0.0019, -0.6008]; % Converted from cm to m
            surface.size = 0.866025; % Converted from cm² to m²
            surface.unit = [0, 0, -1];
        end
        if surfacenum == 3
            surface.bary = [0.4871, -0.0019, 0.2007]; % Converted from cm to m
            surface.size = 0.913944; % Converted from cm² to m²
            surface.unit = [1, 0, 0];
        end
        if surfacenum == 4
            surface.bary = [1.0854, -0.0019, -0.5808]; % Converted from cm to m
            surface.size = 0.690859; % Converted from cm² to m²
            surface.unit = [0, 0, 1];
        end
        if surfacenum == 5
            surface.bary = [1.0854, -0.0019, -0.6008]; % Converted from cm to m
            surface.size = 0.690859; % Converted from cm² to m²
            surface.unit = [0, 0, -1];
        end
        if surfacenum == 6
            surface.bary = [0.2371, 0.4311, 0.2007]; % Converted from cm to m
            surface.size = 0.913944; % Converted from cm² to m²
            surface.unit = [0.5, 0.866, 0];
        end
        if surfacenum == 7
            surface.bary = [0.5362, 0.9492, -0.5808]; % Converted from cm to m
            surface.size = 0.690859; % Converted from cm² to m²
            surface.unit = [0, 0, 1];
        end
        if surfacenum == 8
            surface.bary = [0.5362, 0.9492, -0.6008]; % Converted from cm to m
            surface.size = 0.690859; % Converted from cm² to m²
            surface.unit = [0, 0, -1];
        end
        if surfacenum == 9
            surface.bary = [-0.2629, 0.4311, 0.2007]; % Converted from cm to m
            surface.size = 0.913944; % Converted from cm² to m²
            surface.unit = [-0.5, 0.866, 0];
        end
        if surfacenum == 10
            surface.bary = [-0.5620, 0.9492, -0.5808]; % Converted from cm to m
            surface.size = 0.690859; % Converted from cm² to m²
            surface.unit = [0, 0, 1];
        end
        if surfacenum == 11
            surface.bary = [-0.5620, 0.9492, -0.6008]; % Converted from cm to m
            surface.size = 0.690859; % Converted from cm² to m²
            surface.unit = [0, 0, -1];
        end
        if surfacenum == 12
            surface.bary = [-0.5129, -0.0019, 0.2007]; % Converted from cm to m
            surface.size = 0.913944; % Converted from cm² to m²
            surface.unit = [-1, 0, 0];
        end
        if surfacenum == 13
            surface.bary = [-1.1111, -0.0019, -0.5808]; % Converted from cm to m
            surface.size = 0.690859; % Converted from cm² to m²
            surface.unit = [0, 0, 1];
        end
        if surfacenum == 14
            surface.bary = [-1.1111, -0.0019, -0.6008]; % Converted from cm to m
            surface.size = 0.690859; % Converted from cm² to m²
            surface.unit = [0, 0, -1];
        end
        if surfacenum == 15
            surface.bary = [-0.2629, -0.4349, 0.2007]; % Converted from cm to m
            surface.size = 0.913944; % Converted from cm² to m²
            surface.unit = [-0.5, -0.866, 0];
        end
        if surfacenum == 16
            surface.bary = [-0.5620, -0.9530, -0.5808]; % Converted from cm to m
            surface.size = 0.690859; % Converted from cm² to m²
            surface.unit = [0, 0, 1];
        end
        if surfacenum == 17
            surface.bary = [-0.5620, -0.9530, -0.6008]; % Converted from cm to m
            surface.size = 0.690859; % Converted from cm² to m²
            surface.unit = [0, 0, -1];
        end
        if surfacenum == 18
            surface.bary = [0.2371, -0.4349, 0.2007]; % Converted from cm to m
            surface.size = 0.913944; % Converted from cm² to m²
            surface.unit = [0.5, -0.866, 0];
        end
        if surfacenum == 19
            surface.bary = [0.5362, -0.9530, -0.5808]; % Converted from cm to m
            surface.size = 0.690859; % Converted from cm² to m²
            surface.unit = [0, 0, 1];
        end
        if surfacenum == 20
            surface.bary = [0.5362, -0.9530, -0.6008]; % Converted from cm to m
            surface.size = 0.690859; % Converted from cm² to m²
            surface.unit = [0, 0, -1];
        end
        % 
        bary = R_princ*(surface.bary'); % Barycenter body to princ
        A = (surface.size); % Area in m^2
        N = R_princ*(surface.unit'); % Normal vector in princ
        % 
        % cos_theta_StoN = dot(N,V_p_unit); % Angle between N and V vectors
        theta_StoN = acos(dot(N, V_p_unit));

        % if cos_theta_StoN > 0 % Facing velocity or not 
        %     e = 1;
        % else
        %     e = 0;
        % end

        if theta_StoN >= 0 && theta_StoN <= pi/2
            e = 1; % Surfaces can see each other
        else
            e = 0; % Surfaces are obstructed
        end

        F = -(1/2)*C_d*A*rho*(norm(V_p)^2)*dot(V_p_unit,N)*V_p_unit; % Force
        M_aero = M_aero + cross(bary,F); % Summation 
    end
end

== matlab function main/Orbit Propagation Sun 2.0/Eccentric Anomaly ==
  data: M input; E output; e input; eps input
function E = eccentric_anomaly(M, e, eps)
    M = mod(M,360);
    delta = 2*eps;
    E_i = M;
    E = 2*M;
    while delta > eps
        E = E_i - (E_i - e * sin(E_i) - M)/(1 - e*cos(E_i));
        delta = abs(E - E_i);
        E_i = E;
    end
end

== matlab function main/Orbit Propagation Sun 2.0/Perifocal Coordinates ==
  data: E input; x output; y output; a input; e input
function [x,y] = perifocal_coords(E, a, e)
    x = a*(cos(E) - e);
    y = a * sqrt(1 - e^2) * sin(E);
end

== matlab function main/Orbit Propagation Sun 2.0/oe2ECI ==
  data: nu input; a input; e input; i input; r_ECI output; Om input; om input
function r_ECI =   OE2ECI(nu, a, e, i, Om, om)
    %mu = 398600.435507;

    Rot_Om = [cosd(-Om) sind(-Om) 0;
              -sind(-Om) cosd(-Om) 0
              0 0 1];
    Rot_i = [1 0 0;
            0 cosd(-i) sind(-i);
            0 -sind(-i) cosd(-i)];
    Rot_om = [cosd(-om) sind(-om) 0;
              -sind(-om) cosd(-om) 0
              0 0 1];
    R = Rot_Om * Rot_i * Rot_om;

    
    % Position    
    p = a*(1-e^2);
    r = p/(1+e*cos(nu));
    r_ECI = R * [r*cos(nu); r*sin(nu); 0]; %position vector

end

== matlab function main/Attitude Estimation/Deterministic Attitude Determination ==
  data: M input; V input; DCM_estimated output
%% return sensor measurements
function DCM_estimated = deterministic_attitude_determination(M, V)

    M_fict = M;
    V_fict = V;
    %generate fictitious measurement
    for i = 1:2:length(M(1, :))
        M_fict(:, i) = (M(:, i) + M(:, i+1))./2;
        V_fict(:, i) = (V(:, i) + V(:, i+1))./2;
        M_fict(:, i+1) = (M(:, i) - M(:, i+1))./2;
        V_fict(:, i+1) = (V(:, i) - V(:, i+1))./2;
    end


    DCM_estimated = M_fict * pinv(V_fict); %using fictitous measurements
    %DCM_estimated = M * pinv(V); %no fictitious measurements
        
end

== matlab function main/Orbit Propagation Sun 3.0/Approx ECI ==
  data: time_seconds input; state_sun_ECI output
function state_sun_ECI = our_approxECISunPosition(time_seconds)
% Given Gregorian year(s), day(s), and time(s), calculate Earth-centered
% inertial (ECI) coordinates (in meters) of the vector(s) pointing from
% Earth's center to the center of the Sun.
% Encapsulated by Seth B. Wagenman, from stargazing.net/kepler/sun.html as
% corrected by https://astronomy.stackexchange.com/a/37199/34646 along with
% other minor corrections based on recent revisions to the ecliptic plane.

% Convert seconds since epoch to MATLAB serial date number
time_seconds = squeeze(time_seconds);
MJD = 53029 + time_seconds/86400;
JD = MJD + 2400000.5;

% Convert MJD to datetime
% date_time = datetime(MJD, 'ConvertFrom', 'MJD');
% date_vector = datevec(date_time);


% Extract year, month, day, hour, minute, and second from datetime
% year_val = year(date_time);
% month_val = month(date_time);
% day_val = day(date_time);
% hour_val = hour(date_time);
% minute_val = minute(date_time);
% second_val = second(date_time);

% Create datetime vector
% dateTimeVector = [year_val, month_val, day_val, hour_val, minute_val, second_val];

% Set time(s) relative to the J2000.0 epoch
fractionalDay = JD - 2451545.0;

% Mean longitude of the Sun
meanLongitudeSunDegrees = 280.4606184 + ...
	((36000.77005361 / 36525) * fractionalDay); %(degrees)

% Mean anomaly of the Sun
meanAnomalySunDegrees = 357.5277233 + ...
	((35999.05034 / 36525) * fractionalDay); %(degrees)
meanAnomalySunRadians = meanAnomalySunDegrees * pi / 180;

% Ecliptic longitude of the Sun
eclipticLongitudeSunDegrees = meanLongitudeSunDegrees + ...
	(1.914666471 * sin(meanAnomalySunRadians)) + ...
	(0.918994643 * sin(2 * meanAnomalySunRadians)); %(degrees)
eclipticLongitudeSunRadians = eclipticLongitudeSunDegrees * pi / 180;

% Obliquity of the ecliptic plane formula mostly derived from:
% https://en.wikipedia.org/wiki/Ecliptic#Obliquity_of_the_ecliptic
epsilonDegrees = ... % Formula deals with time denominated in centuries
	23.43929 - ((46.8093 / 3600) * fractionalDay / 36525);  %(degrees)
epsilonRadians = epsilonDegrees * pi / 180;

% **** Calculations for unit vectors direction to the Sun are in ECI ****
% Now calculate the Earth to Sun unit vector(s) USING RADIANS, NOT DEGREES
unitEarthSunVectorTransposed = [cos(eclipticLongitudeSunRadians).';
    (cos(epsilonRadians) .* sin(eclipticLongitudeSunRadians)).';
    (sin(epsilonRadians) .* sin(eclipticLongitudeSunRadians)).'];
unitEarthSunVector = unitEarthSunVectorTransposed.';

% Scale up from unit vector(s); distances vary--Earth's orbit is elliptical
distEarthToSunInAstronomicalUnits = ...
	1.000140612 - ...
	(0.016708617 * cos(meanAnomalySunRadians)) - ...
	(0.000139589 * cos(2 * meanAnomalySunRadians)); % in Astronomical Units
distEarthToSunInMeters = ... % (new international definition for an A. U.)
	149597870700 * distEarthToSunInAstronomicalUnits;

% Multiply unit vector(s) by distance to Sun for scaling to full magnitude
state_sun_ECI = ... % Use meters for generic code compatibility
	(distEarthToSunInMeters .* unitEarthSunVector)/1000; 

end % End of function

== matlab function main/Attitude Estimation/MATLAB Function ==
  data: M input; quat_estimated output; V input
%% return estimated quaternions M = sun, magnet, star1, star2
function quat_estimated = Q_method(M, V)
    w_sun = 0.1;
    w_mag = 0.05;
    w_star = 0.85;
    W = M;
    W(:,3:end) = sqrt(w_star).*M(:,3:end);
    W(:, 2) = sqrt(w_mag) .*M(:, 2);
    W(:, 1) = sqrt(w_sun) .*M(:, 1);

    U = V;
    U(:,3:end) = sqrt(w_star).*V(:,3:end);
    U(:, 2) = sqrt(w_mag) .*V(:, 2);
    U(:, 1) = sqrt(w_sun) .*V(:, 1);
 

    B = W*U';
    S = B + B';
    Z = [B(2,3) - B(3,2); B(3,1) - B(1,3); B(1,2)-B(2,1)];

    sigma = trace(B);

    K = [S - sigma*eye(3), Z; Z', sigma];
    [eigvec, eigval] = eig(K);
    eigenvalues = diag(eigval);

    [max_eigenvalue, max_index] = max(eigenvalues);

    max_eigvec = eigvec(:, max_index);

    quat_estimated = [real(max_eigvec(1)); real(max_eigvec(2)); real(max_eigvec(3)); real(max_eigvec(4))];
    quat_estimated = quat_estimated./norm(quat_estimated);
end

== matlab function main/Environment Petrubations/Compute Air Density/MATLAB Function ==
  data: r_ECI input; geodetic output
function geodetic = fcn(r_ECI)
    rE = 6378;
    h = norm(r_ECI) - rE;
    lat = atan2(r_ECI(3), sqrt(r_ECI(1)^2 + r_ECI(2)^2));
    long = atan2(r_ECI(2), r_ECI(1));
    geodetic = [lat, long, h*1000];
end

== matlab function main/Attitude Estimation/Quaternions/Initial Quaternions ==
  data: C input; quaternions_init output
%% Quaternions
function quaternions_init = inital_quaternions(C)
    beta_4sq = (0.25*(1+trace(C)));
    beta_1sq = (0.25*(1+2*C(1,1)- trace(C)));
    beta_2sq = (0.25*(1+2*C(2,2)- trace(C)));
    beta_3sq = (0.25*(1+2*C(3,3)- trace(C)));
    
    [maximum, max_ind] = max([beta_1sq, beta_2sq, beta_3sq, beta_4sq]);
    
    switch max_ind
        case 1
            beta_1 = sqrt(beta_1sq);
            beta_4 = (C(2,3) - C(3,2))/(4*beta_1);
            beta_3 = (C(3,1) + C(1,3))/(4*beta_1);
            beta_2 = (C(1,2) + C(2,1))/(4*beta_1);
        case 2
            beta_2 = sqrt(beta_2sq);
            beta_4 = (C(3,1) - C(1,3))/(4*beta_2);
            beta_3 = (C(2,3) + C(3,2))/(4*beta_2);
            beta_1 = (C(1,2) + C(2,1))/(4*beta_2);
        case 3
            beta_3 = sqrt(beta_3sq);
            beta_4 = (C(1,2) - C(2,1))/(4*beta_3);
            beta_2 = (C(2,3) + C(3,2))/(4*beta_3);
            beta_1 = (C(3,1) + C(1,3))/(4*beta_3);
           
        otherwise
            beta_4 = sqrt(beta_4sq);
            beta_3 = (C(1,2) - C(2,1))/(4*beta_4);
            beta_2 = (C(3,1) - C(1,3))/(4*beta_4);
            beta_1 = (C(2,3) - C(3,2))/(4*beta_4);   
    end
    
    quaternions_init = [beta_1; beta_2; beta_3; beta_4];
    quaternions_init =  quaternions_init/ norm(quaternions_init); %normalize
end

== matlab function main/Attitude Estimation/Quaternions/Kinematic Equations Quaternions  ==
  data: omega input; quaternion input; quat_dot output
%% Kinematic Equation of motion quaternions
function quat_dot = quaternions_dot(omega, quaternion)
    Sigma = [0, omega(3), -omega(2), omega(1);
            -omega(3), 0, omega(1), omega(2);
            omega(2), -omega(1), 0, omega(3);
            -omega(1), -omega(2), -omega(3), 0];
    quat_dot = 0.5 * Sigma * quaternion;
end

== matlab function main/Spacecraft Subsystem/Measurement Generation ==
  data: sunsensor output; Rot input; sunsensor_gt input; rand_sun input; magnetometer_gt input; rand_magnet input; startracker_1_gt input; startracker_2_gt input; rand_star input; magnetometer output; startracker_1 output; startracker_2 output
%% return sensor measurements from ground truth

function [sunsensor, magnetometer, startracker_1, startracker_2] = measurement_generation(Rot, sunsensor_gt, rand_sun, magnetometer_gt, rand_magnet, startracker_1_gt, startracker_2_gt, rand_star)
    magnetometer = Rot * magnetometer_gt;
    magnetometer = [magnetometer(1)*(1+rand_magnet(1)); magnetometer(2)*(1+rand_magnet(2)); magnetometer(3)*(1+rand_magnet(3))];
    sunsensor = Rot*sunsensor_gt;
    sunsensor =   rotationMatrix_z(rand_sun(1))*rotationMatrix(cross([sunsensor(1:2);0], [0; 0;1]), rand_sun(2))*sunsensor;
    startracker_1 = Rot * startracker_1_gt;
    startracker_2 = Rot * startracker_2_gt;
    for i = 1:length(startracker_1(1,:))
       startracker_1(:, i) = rotationMatrix_z(rand_star(1, i))*rotationMatrix(cross([startracker_1(1:2, i);0], [0; 0;1]), rand_star(2, i))*startracker_1(:, i);
       startracker_2(:, i) = rotationMatrix_z(rand_star(3, i))*rotationMatrix(cross([startracker_2(1:2, i);0], [0; 0;1]), rand_star(4, i))*startracker_2(:, i);
    end


end
function R = rotationMatrix(axis, angle)
    axis = axis ./ norm(axis);
    x = axis(1);
    y = axis(2);
    z = axis(3);
    c = cosd(angle);
    s = sind(angle);
    t = 1 - c;

    R = [t*x*x + c,    t*x*y - s*z,  t*x*z + s*y;
         t*x*y + s*z,  t*y*y + c,    t*y*z - s*x;
         t*x*z - s*y,  t*y*z + s*x,  t*z*z + c];
end

function R_z = rotationMatrix_z(angle)
    c = cosd(angle);
    s = sind(angle);
    
    % Construct the rotation matrix around the z-axis
    R_z = [c, -s, 0;
         s,  c, 0;
         0,  0, 1];
end

== matlab function main/Spacecraft Subsystem/Reference Truth ==
  data: sunsensor output; magnetometer output; Rot input; magnetic_field input; r_sun input; startracker_1 output; startracker_2 output
%% return ground truth in ECI
function [sunsensor,  magnetometer, startracker_1, startracker_2] = reference_truth(Rot, magnetic_field, r_sun)
    magnetometer = Rot'*magnetic_field; 
    sunsensor = r_sun(1:3)./norm(r_sun(1:3)); %already in ECI
    startracker_1 = zeros(3, 15);
    startracker_2 = zeros(3, 15);
    for i = 1:length(startracker_1(1,:))
        RA1 = 75 + i;
        declination1 = 35 + i;
        startracker_1(:, i) = Rot'*[cosd(RA1)*cosd(declination1); sind(RA1)*cosd(declination1); sind(declination1)]; %target for body z-axis
        RA2 = 250 + i;
        declination2 = 12 + i;
        startracker_2(:, i) = Rot'*[cosd(RA2)*cosd(declination2); sind(RA2)*cosd(declination2); sind(declination2)]; %target for body z-axis
    end
end

== matlab function main/Attitude Estimation/EKF time update ==
  data: x_prev input; x0 input; P0 input; inertia_p input; del_t input; x_post_min output; P_prev input; P_post_min output
function [x_post_min, P_post_min] = EKF_time_update(x_prev, x0, P0, inertia_p, del_t, P_prev)
    wx = x_prev(1);
    wy = x_prev(2);
    wz = x_prev(3);
    q1 = x_prev(4);
    q2 = x_prev(5);
    q3 = x_prev(6);
    q4 = x_prev(7);

    if (isempty(x_prev)) %for initialization
        x_prev = x0;
        P_prev = P0;
    end

    om = norm(x_prev(1:3));
    k = 1/om * sin(om * del_t/2);
    phi = zeros([7,7]); %state transition matrix
    phi(1:3, 1:3) = [1, (inertia_p(2,2) - inertia_p(3,3))/inertia_p(1,1) * x_prev(3)*del_t, (inertia_p(2,2) - inertia_p(3,3))/inertia_p(1,1) * x_prev(2)*del_t;
        (inertia_p(3,3) -inertia_p(1,1))/inertia_p(2,2) * x_prev(3) * del_t, 1, (inertia_p(3,3) -inertia_p(1,1))/inertia_p(2,2) * x_prev(1) * del_t;
        (inertia_p(1,1) -inertia_p(2,2))/inertia_p(3,3) * x_prev(2) * del_t, (inertia_p(1,1) -inertia_p(2,2))/inertia_p(3,3) * x_prev(1) * del_t, 1];
    phi(4:end, :) = [k*q4, -k*q3, k*q2, cos(om*del_t/2), k*wz, -k*wy, k*wx;
                    k*q3, k*q4, -k*q1, -k*wz, cos(om*del_t/2), k*wx, k*wy;
                    -k*q2, k*q1, k*q4, k*wy, -k*wx, cos(om*del_t/2), k*wz;
                    -k*q1, -k*q2, -k*q3, -k*wx, -k*wy, -k*wz, cos(om*del_t/2)];


    Q = 1/100 .* eye(7); %process noise
    x_post_min = phi * x_prev;
    P_post_min = phi * P_prev * phi' + Q;

== matlab function main/Quaternions/Kinematic Equations Quaternions  ==
  data: omega input; quaternion input; quat_dot output
%% Kinematic Equation of motion quaternions
function quat_dot = quaternions_dot(omega, quaternion)
    Sigma = [0, omega(3), -omega(2), omega(1);
            -omega(3), 0, omega(1), omega(2);
            omega(2), -omega(1), 0, omega(3);
            -omega(1), -omega(2), -omega(3), 0];
    quat_dot = 0.5 * Sigma * quaternion;
end
